simulink model "lab_harmonic_mdl"  (R2023a)
settings: Solver=VariableStepAuto  StartTime=0.0  StopTime=10.0  RelTol=1e-3
settings Model: Creator=gnomy  LastModifiedBy=gnomy

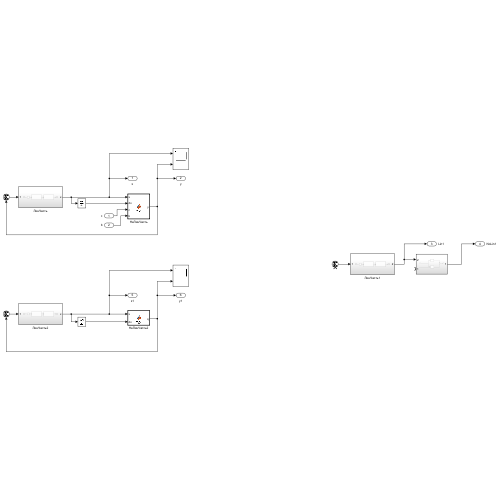
[thumbnail: Simulink's stored preview of the top-level diagram]
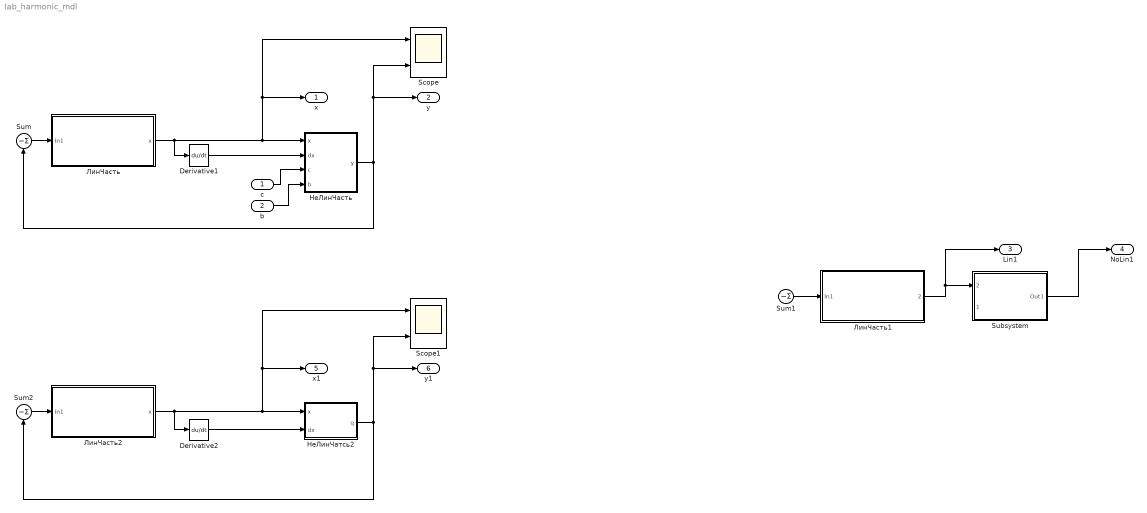
== system lab_harmonic_mdl ==
  c : Inport
  b : Inport  Port=2
  Derivative1 : Derivative
  Derivative2 : Derivative
  Scope : Scope  NumInputPorts=2
  Scope1 : Scope  NumInputPorts=2
  Subsystem : Subsystem
  Sum : Sum  Inputs=||-
  Sum1 : Sum  Inputs=||-
  Sum2 : Sum  Inputs=||-
  ЛинЧасть : Subsystem
  ЛинЧасть1 : Subsystem
  ЛинЧасть2 : Subsystem
  НеЛинЧасть : MATLAB Function  TreatAsAtomicUnit=on
  НеЛинЧатсь2 : MATLAB Function  TreatAsAtomicUnit=on
  x : Outport
  y : Outport  Port=2
  Lin1 : Outport  Port=3
  NoLin1 : Outport  Port=4
  x1 : Outport  Port=5
  y1 : Outport  Port=6
  wires:
  Sum/1 -> ЛинЧасть/1(In1)
  ЛинЧасть/1(x) -> Derivative1/1, Scope/1, x/1, НеЛинЧасть/1(x)
  НеЛинЧасть/1(y) -> Sum/1, Scope/2, y/1
  c/1 -> НеЛинЧасть/3(c)
  b/1 -> НеЛинЧасть/4(b)
  Subsystem/1(Out1) -> NoLin1/1
  ЛинЧасть1/1(2) -> Lin1/1, Subsystem/1(2)
  Sum1/1 -> ЛинЧасть1/1(In1)
  Derivative1/1 -> НеЛинЧасть/2(dx)
  НеЛинЧатсь2/1(q) -> Scope1/2, y1/1, Sum2/1
  ЛинЧасть2/1(x) -> Derivative2/1, Scope1/1, x1/1, НеЛинЧатсь2/1(x)
  Sum2/1 -> ЛинЧасть2/1(In1)
  Derivative2/1 -> НеЛинЧатсь2/2(dx)

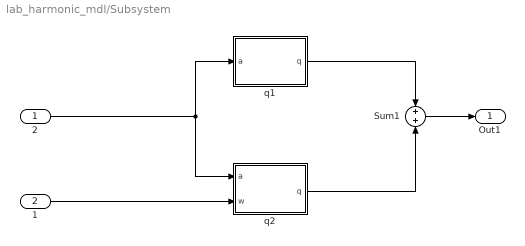
== system lab_harmonic_mdl/Subsystem ==
  2 : Inport
  1 : Inport  Port=2
  Sum1 : Sum  Inputs=+|+
  q1 : MATLAB Function  TreatAsAtomicUnit=on
  q2 : MATLAB Function  TreatAsAtomicUnit=on
  Out1 : Outport
  wires:
  q2/1(q) -> Sum1/2
  q1/1(q) -> Sum1/1
  Sum1/1 -> Out1/1
  2/1 -> q2/1(a), q1/1(a)
  1/1 -> q2/2(w)

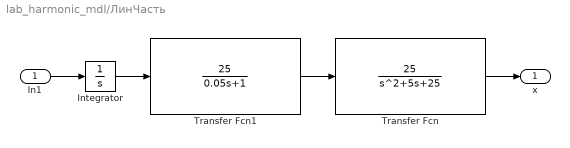
== system lab_harmonic_mdl/ЛинЧасть ==
  In1 : Inport
  Integrator : Integrator
  Transfer Fcn : TransferFcn  Numerator=[25]  Denominator=[1 5 25]
  Transfer Fcn1 : TransferFcn  Numerator=[25]  Denominator=[0.05 1]
  x : Outport
  wires:
  In1/1 -> Integrator/1
  Transfer Fcn/1 -> x/1
  Transfer Fcn1/1 -> Transfer Fcn/1
  Integrator/1 -> Transfer Fcn1/1

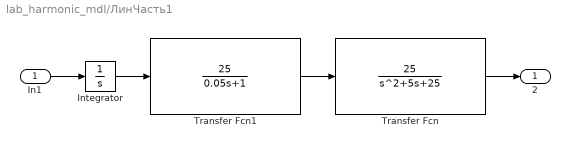
== system lab_harmonic_mdl/ЛинЧасть1 ==
  In1 : Inport
  Integrator : Integrator
  Transfer Fcn : TransferFcn  Numerator=[25]  Denominator=[1 5 25]
  Transfer Fcn1 : TransferFcn  Numerator=[25]  Denominator=[0.05 1]
  2 : Outport
  wires:
  In1/1 -> Integrator/1
  Transfer Fcn/1 -> 2/1
  Transfer Fcn1/1 -> Transfer Fcn/1
  Integrator/1 -> Transfer Fcn1/1

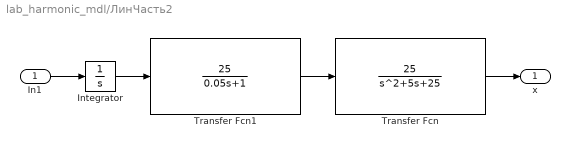
== system lab_harmonic_mdl/ЛинЧасть2 ==
  In1 : Inport
  Integrator : Integrator
  Transfer Fcn : TransferFcn  Numerator=[25]  Denominator=[1 5 25]
  Transfer Fcn1 : TransferFcn  Numerator=[25]  Denominator=[0.05 1]
  x : Outport
  wires:
  In1/1 -> Integrator/1
  Transfer Fcn/1 -> x/1
  Transfer Fcn1/1 -> Transfer Fcn/1
  Integrator/1 -> Transfer Fcn1/1

== matlab function lab_harmonic_mdl/НеЛинЧасть ==
  data: x input; dx input; y output; c input; b input
function y  = rele(x, dx, c, b)
    
    if ode45(x)
        y = c*sign(x-b); 
    else
        y = c*sign(x+b);
    end

end

== matlab function lab_harmonic_mdl/Subsystem/q1 ==
  data: a input; q output
function q  = q1(a)

    c = 1;
    b = 1;

    q = sqrt(1 - (b^2 / a^2)) * (4*c)/(pi*a);

end

== matlab function lab_harmonic_mdl/Subsystem/q2 ==
  data: a input; q output; w input
function q  = q2(a, w)

    c = 1;
    b = 1;

    q = -(4*c*b)/(w*pi*a^2);

end

== matlab function lab_harmonic_mdl/НеЛинЧатсь2 ==
  data: x input; q output; dx input
function q  = W3(x, dx)

    c = 1;
    b = 1;

    q = sqrt(1 - (b^2 / a^2)) * (4*c)/(pi*a);

end
